simulink model "slip_air"  (R2019a)
settings: Solver=VariableStepAuto  StartTime=0.0  StopTime=ta  RelTol=1e-1
values from neighbouring files (symbols this model uses):
  g = -9.81    [SLIP.m]    (also in SLIP_alfa0.m; slipFarley93.m)
  L0 = Lhk + Lkf    (= 0.56)    [SLIP.m]    (also in SLIP_alfa0.m; slipFarley93.m)
  Lcol = 0.70    (= 0.7)    [SLIP.m]
  M = 15+3    (= 18)    [SLIP.m]    (also in SLIP_alfa0.m; slipFarley93.m)
  vxSlipfinal = vxSlip( length(toutSlip) )    [SLIP.m]    (also in SLIP_alfa0.m = vxSlip( length(vxSlip) ); slipFarley93.m = vxSlip( length(vxSlip) ))
  vySlipfinal = vySlip( length(toutSlip) )    [SLIP.m]    (also in SLIP_alfa0.m = vySlip( length(vySlip) ); slipFarley93.m = vySlip( length(vySlip) ))
  xSlipfinal = xSlip( length(toutSlip) )    [SLIP.m]    (also in SLIP_alfa0.m = xSlip( length(xSlip) ); slipFarley93.m = xSlip( length(xSlip) ))
  ySlipfinal = ySlip( length(toutSlip) )    [SLIP.m]    (also in SLIP_alfa0.m = ySlip( length(ySlip) ); slipFarley93.m = ySlip( length(ySlip) ))
settings Model: Creator=Jesus  LastModifiedBy=Jesus

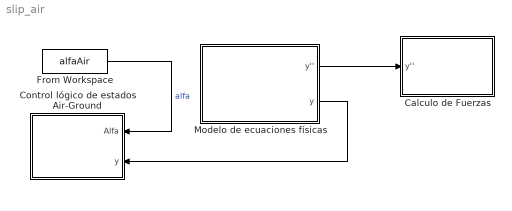
== system slip_air ==
  Calculo de Fuerzas : Subsystem
  Control lógico de estados Air-Ground : Subsystem
  From Workspace : FromWorkspace  VariableName=alfaAir  SampleTime=0
  Modelo de ecuaciones físicas : Subsystem
  wires:
  From Workspace/1 -> Control lógico de estados Air-Ground/1(Alfa)  "alfa"
  Modelo de ecuaciones físicas/2(y) -> Control lógico de estados Air-Ground/2(y)
  Modelo de ecuaciones físicas/1(y'') -> Calculo de Fuerzas/1(y'')

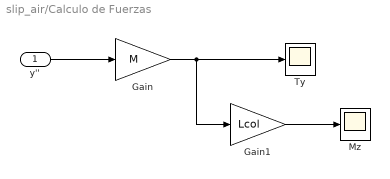
== system slip_air/Calculo de Fuerzas ==
  y'' : Inport
  Gain : Gain  Gain=M
  Gain1 : Gain  Gain=Lcol
  Mz : Scope
  Ty : Scope
  wires:
  y''/1 -> Gain/1
  Gain/1 -> Gain1/1, Ty/1
  Gain1/1 -> Mz/1

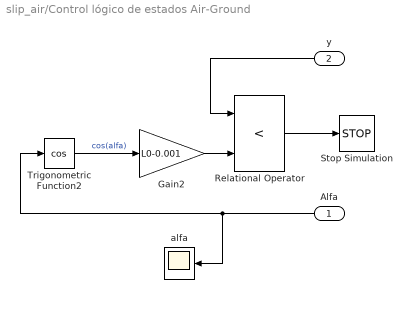
== system slip_air/Control lógico de estados Air-Ground ==
  Alfa : Inport
  y : Inport  Port=2
  Gain2 : Gain  Gain=L0-0.001
  Relational Operator : RelationalOperator  Operator=<  OutDataTypeStr=boolean  RndMeth=Simplest
  Stop Simulation : Stop
  Trigonometric Function2 : Trigonometry  Operator=cos
  alfa : Scope
  wires:
  Trigonometric Function2/1 -> Gain2/1  "cos(alfa)"
  Relational Operator/1 -> Stop Simulation/1
  Gain2/1 -> Relational Operator/2
  Alfa/1 -> alfa/1, Trigonometric Function2/1
  y/1 -> Relational Operator/1

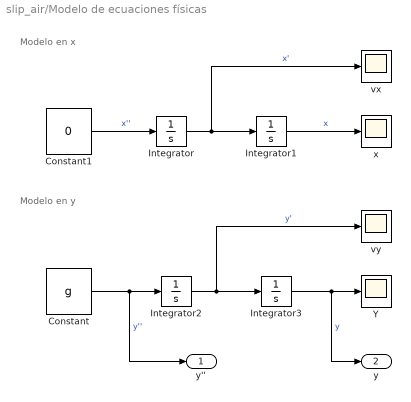
== system slip_air/Modelo de ecuaciones físicas ==
  note: Modelo en x
  note: Modelo en y
  Constant : Constant  Value=g
  Constant1 : Constant  Value=0
  Integrator : Integrator  InitialCondition=vxSlipfinal
  Integrator1 : Integrator  InitialCondition=xSlipfinal
  Integrator2 : Integrator  InitialCondition=vySlipfinal
  Integrator3 : Integrator  InitialCondition=ySlipfinal
  Y : Scope
  vx : Scope
  vy : Scope
  x : Scope
  y'' : Outport
  y : Outport  Port=2
  wires:
  Integrator2/1 -> vy/1, Integrator3/1  "y'"
  Integrator/1 -> vx/1, Integrator1/1  "x'"
  Integrator3/1 -> Y/1, y/1  "y"
  Integrator1/1 -> x/1  "x"
  Constant/1 -> y''/1, Integrator2/1  "y''"
  Constant1/1 -> Integrator/1  "x''"
